simulink model "izhikevichTest"  (R2020b)
settings: Solver=FixedStepAuto  StartTime=0.0  StopTime=0.5  FixedStep=0.001  RelTol=1e-3
libraries: simulink x2
settings Model: EnablePacing=on  PacingRate=0.071000  Creator=40129232  LastModifiedBy=adamalcorn
settings SolverCC: AlgebraicLoopSolver=LineSearch
settings DataIOCC: ReturnWorkspaceOutputs=off
settings OptimizationCC: LifeSpan=inf
settings DebuggingCC: SFExecutionAtInitializationDiag=none  ArithmeticOperatorsInVariantConditions=warning
settings SFSimCC: SimUseLocalCustomCode=off  CustomCodeUndefinedFunction=UseInterfaceOnly
settings RTWCC: RTWUseLocalCustomCode=off
settings CodeAppCC: StateflowObjectComments=on

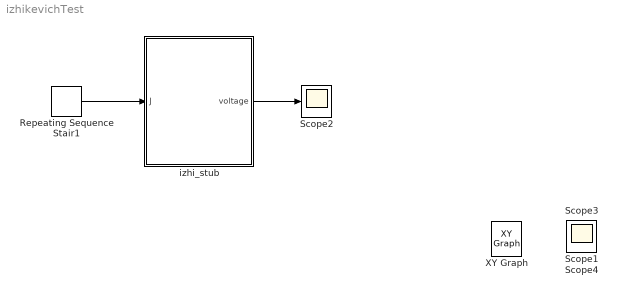
== system izhikevichTest ==
  Repeating Sequence Stair1 : simulink/Sources/Repeating Sequence Stair  OutValues=[40.37, 52.35, 62.17, 70.19, 76.75].'  tsamp=-1  OutMin=[]  OutMax=[]  OutDataTypeStr=double  OutputDataTypeScalingMode=double  OutDataType=fixdt(0,8)  ConRadixGroup=Best Precision: Vector-wise  OutScaling=2^-12
  Scope{1..4} (4 alike) : Scope
  izhi_stub : Subsystem
  XY Graph : simulink/Sinks/XY Graph  IOType=viewer  xmin=-1  xmax=1  ymin=-1  ymax=1  st=-1
  wires:
  Repeating Sequence Stair1/1 -> izhi_stub/1(J)
  izhi_stub/1(voltage) -> Scope2/1

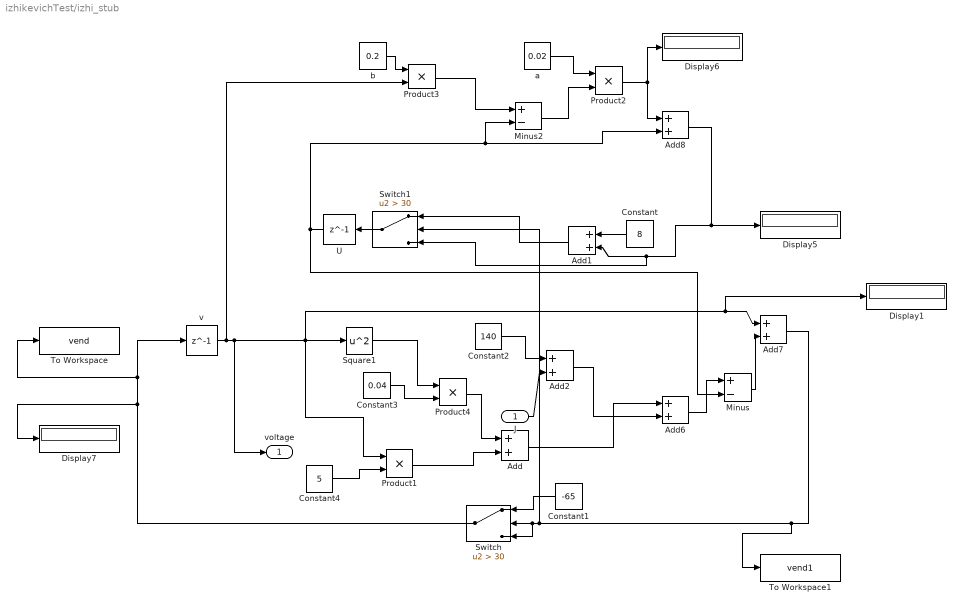
== system izhikevichTest/izhi_stub ==
  J : Inport
  Add{,1..2,6..8} (6 alike) : Sum
  Constant : Constant  Value=8
  Constant1 : Constant  Value=-65
  Constant2 : Constant  Value=140
  Constant3 : Constant  Value=0.04
  Constant4 : Constant  Value=5
  Display{1,5..7} (4 alike) : Display
  Minus : Sum  Inputs=+-
  Minus2 : Sum  Inputs=+-
  Product{1..4} (4 alike) : Product
  Square1 : Math  Operator=square  SaturateOnIntegerOverflow=on
  Switch : Switch  Criteria=u2 > Threshold  Threshold=30
  Switch1 : Switch  Criteria=u2 > Threshold  Threshold=30
  To Workspace : ToWorkspace  VariableName=vend  SaveFormat=Timeseries  SampleTime=-1
  To Workspace1 : ToWorkspace  VariableName=vend1  SaveFormat=Timeseries  SampleTime=-1
  U : Delay  DelayLength=1  InitialCondition=0
  a : Constant  Value=0.02
  b : Constant  Value=0.2
  v : Delay  DelayLength=1  InitialCondition=-65
  voltage : Outport  VectorParamsAs1DForOutWhenUnconnected=off
  wires:
  Product1/1 -> Add/2
  Product4/1 -> Add/1
  Product2/1 -> Add8/1, Display6/1
  J/1 -> Add2/2
  Constant1/1 -> Switch/1
  Constant/1 -> Add1/1
  Add1/1 -> Switch1/1
  Add/1 -> Add6/1
  Switch1/1 -> U/1
  Add2/1 -> Add6/2
  Constant2/1 -> Add2/1
  b/1 -> Product3/1
  Switch/1 -> v/1, To Workspace/1, Display7/1
  U/1 -> Add8/2, Minus2/2, Minus/2
  a/1 -> Product2/1
  Minus2/1 -> Product2/2
  Add8/1 -> Switch1/3, Add1/2, Display5/1
  Constant4/1 -> Product1/2
  Square1/1 -> Product4/1
  Constant3/1 -> Product4/2
  Add7/1 -> To Workspace1/1, Switch1/2, Switch/3, Switch/2
  Product3/1 -> Minus2/1
  Add6/1 -> Minus/1
  Minus/1 -> Add7/2
  v/1 -> Product3/2, voltage/1, Square1/1, Display1/1, Add7/1, Product1/1
